simulink model "AlphaBot_Control_Loop"  (R2023a)
settings: Solver=ode45  StartTime=0.0  StopTime=10  RelTol=1e-3
libraries: slpidlib x1
settings Model: Creator=hshl-user  LastModifiedBy=hshl-user

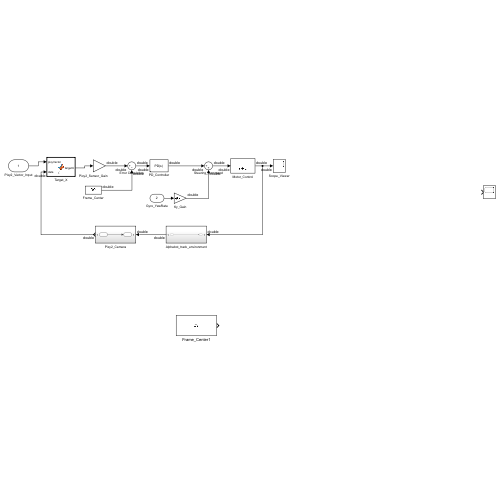
[thumbnail: Simulink's stored preview of the top-level diagram]
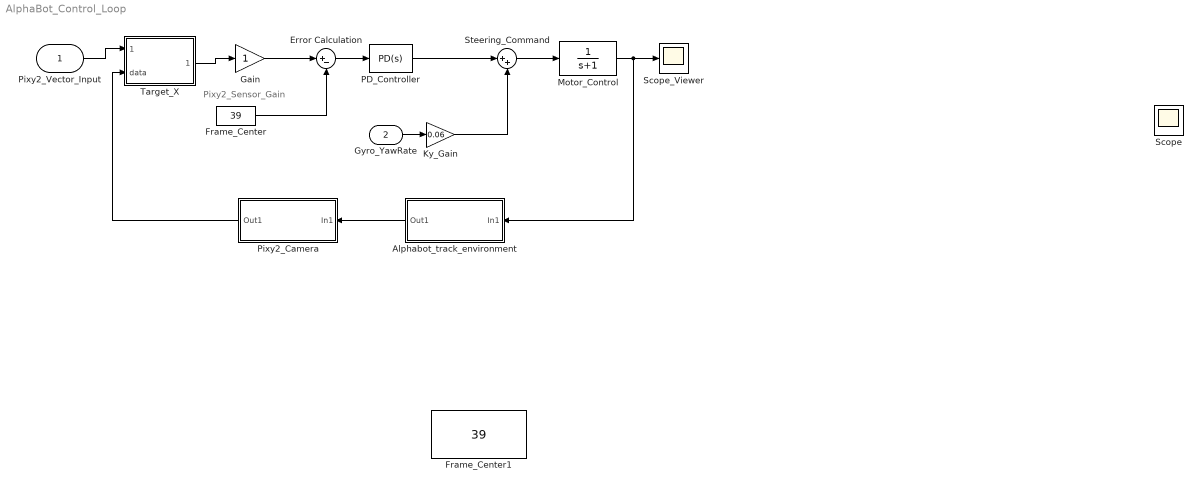
== system AlphaBot_Control_Loop ==
  note: Pixy2_Sensor_Gain
  Pixy2_Vector_Input : Inport
  Gyro_YawRate : Inport  Port=2
  Alphabot_track_environment : Subsystem
  Error Calculation : Sum  Inputs=|+-
  Frame_Center : Constant  Value=39
  Frame_Center1 : Constant  Value=39
  Gain : Gain
  Ky_Gain : Gain  Gain=0.06
  Motor_Control : TransferFcn  Denominator=[1 1]
  PD_Controller : slpidlib/PID Controller  Controller=PD  Form=Parallel  TimeDomain=Continuous-time  UseExternalTs=off  SampleTime=-1  IntegratorMethod=Forward Euler  FilterMethod=Forward Euler  ControllerParametersSource=internal  P=6.8  I=1  UseKiTs=off  D=4.0  N=100  UseFilter=on  TunerSelectOption=Transfer Function Based (PID Tuner App)  InitialConditionSource=internal  InitialConditionForIntegrator=0  InitialConditionForFilter=0  DifferentiatorICPrevScaledInput=0  ExternalReset=none  TrackingMode=off  Kt=1  LimitOutput=off  SatLimitsSource=internal  UpperSaturationLimit=inf  LowerSaturationLimit=-inf  LinearizeAsGain=on  AntiWindupMode=none  Kb=1  LimitIntegrator=off  UpperIntegratorSaturationLimit=inf  LowerIntegratorSaturationLimit=-inf  POutMin=[]  POutMax=[]  IOutMin=[]  IOutMax=[]  DOutMin=[]  DOutMax=[]  NOutMin=[]  NOutMax=[]  SumOutMin=[]  SumOutMax=[]  SaturationOutMin=[]  SaturationOutMax=[]  PParamMin=[]  PParamMax=[]  IParamMin=[]  IParamMax=[]  DParamMin=[]  DParamMax=[]  NParamMin=[]  NParamMax=[]  KbParamMin=[]  KbParamMax=[]  KtParamMin=[]  KtParamMax=[]  KbOutMin=[]  KbOutMax=[]  KtOutMin=[]  KtOutMax=[]  IntegratorOutMin=[]  IntegratorOutMax=[]  FilterOutMin=[]  FilterOutMax=[]  SumI1OutMin=[]  SumI1OutMax=[]  SumI2OutMin=[]  SumI2OutMax=[]  SumI3OutMin=[]  SumI3OutMax=[]  SumI4OutMin=[]  SumI4OutMax=[]  SumDOutMin=[]  SumDOutMax=[]  DifferentiatorOutMin=[]  DifferentiatorOutMax=[]  FilterDiffOutCoefMin=[]  FilterDiffOutCoefMax=[]  ReciprocalOutMin=[]  ReciprocalOutMax=[]  SumDenOutMin=[]  SumDenOutMax=[]  SumNumOutMin=[]  SumNumOutMax=[]  DivideOutMin=[]  DivideOutMax=[]  UdiffTsProdOutMin=[]  UdiffTsProdOutMax=[]  NTsProdOutMin=[]  NTsProdOutMax=[]  UintegralTsProdOutMin=[]  UintegralTsProdOutMax=[]  UngainTsProdOutMin=[]  UngainTsProdOutMax=[]  ClampingZeroOutDataTypeStr=Inherit: Inherit via back propagation  ClampingZeroOutMin=[]  ClampingZeroOutMax=[]  FilterDenConstantOutDataTypeStr=Inherit: Inherit via back propagation  FilterDenConstantOutMin=[]  FilterDenConstantOutMax=[]  PCopyOutDataTypeStr=Inherit: Inherit via back propagation  PCopyOutMin=[]  PCopyOutMax=[]  NCopyOutDataTypeStr=Inherit: Inherit via back propagation  NCopyOutMin=[]  NCopyOutMax=[]  IntegratorContinuousStateAttributes=''  IntegratorStateMustResolveToSignalObject=off  IntegratorRTWStateStorageClass=Auto  FilterContinuousStateAttributes=''  FilterStateMustResolveToSignalObject=off  FilterRTWStateStorageClass=Auto  ParallelPVariant=InternalParameters  IdealPVariant=Disabled  IVariant=Disabled  DVariant=InternalParameters  IntegratorVariant=Disabled  SatVariant=Disabled  AWVariant=Disabled  PCopyVariant=Disabled  TRVariant=Disabled  FdbkBlocksVariant=Forward  IdealPFdbkVariant=Disabled  SatFdbkVariant=Disabled  DerivativeFilterVariant=ContFilter  NVariant=InternalParameters  NCopyVariant=Disabled  FilterICVariant=InternalICsFilter  IntegratorICVariant=Disabled  ExternalResetVariant=Disabled  TRSumVariant=Passthrough  SumFdbkVariant=Disabled  SumVariant=Sum_PD  TsampFilterVariant=InternalTs  TsampNgainVariant=Passthrough  TsampIntegralVariant=Disabled_SignalSpec  ExternalSaturationOutDataTypeStr=Inherit: Same as second input
  Pixy2_Camera : Subsystem
  Scope : Scope
  Scope_Viewer : Scope
  Steering_Command : Sum  Inputs=|++
  Target_X : MATLAB Function  TreatAsAtomicUnit=on
  wires:
  Motor_Control/1 -> Alphabot_track_environment/1(In1), Scope_Viewer/1
  Gyro_YawRate/1 -> Ky_Gain/1
  Error Calculation/1 -> PD_Controller/1
  Frame_Center/1 -> Error Calculation/2
  PD_Controller/1 -> Steering_Command/1
  Steering_Command/1 -> Motor_Control/1
  Ky_Gain/1 -> Steering_Command/2
  Pixy2_Vector_Input/1 -> Target_X/1(pixyVector)
  Target_X/1(targetX) -> Gain/1
  Gain/1 -> Error Calculation/1
  Alphabot_track_environment/1(Out1) -> Pixy2_Camera/1(In1)
  Pixy2_Camera/1(Out1) -> Target_X/2(data)

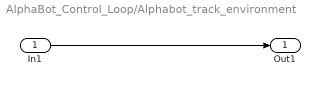
== system AlphaBot_Control_Loop/Alphabot_track_environment ==
  In1 : Inport
  Out1 : Outport
  wires:
  In1/1 -> Out1/1

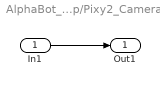
== system AlphaBot_Control_Loop/Pixy2_Camera ==
  In1 : Inport
  Out1 : Outport
  wires:
  In1/1 -> Out1/1

== matlab function AlphaBot_Control_Loop/Target_X ==
  data: pixyVector input; targetX output; data input
function targetX = fcn(pixyVector, data)

x0 = pixyVector(1);
x1 = pixyVector(3);

targetX = (x0 + x1) / 2;
end
